simulink library "sm_trackV_lib_terrain_contact_s45"  (R2026a)
settings: Solver=VariableStepAuto
undefined symbols (not defined in the file): L1, L10, L11, L12, L13, L14, L15, L16, L17, L18, L19, L2, L20, L21, L22, L23, L24, L25, L26, L27, L28, L29, L3, L30, L31, L32, L33, L34, L35, L36, L37, L38, L39, L4, L40, L41, L42, L43, L44, L45, L5, L6, L7, L8, L9, Scene, X, Y, Z
libraries: sm_trackV_lib_terrain_contact_elem x45, $bdroot x19, sm_lib x12, sm_excv_scene_lib x3
Description:
  | Copyright 2024-2026 The MathWorks, Inc.
settings Model: Creator=smiller  LastModifiedBy=smiller

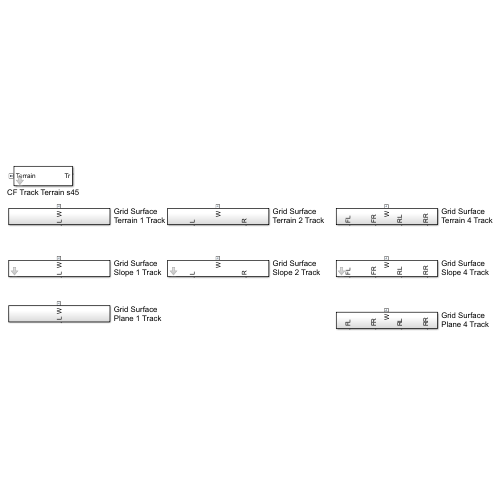
[thumbnail: Simulink's stored preview of the top-level diagram]
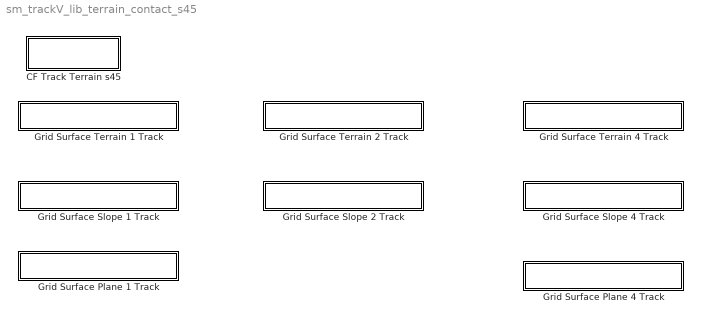
== system sm_trackV_lib_terrain_contact_s45 ==
  CF Track Terrain s45 : Subsystem  mask(Contact Forces, Full Track to Terrain){K_Road=Scene.Contact.Terrain.K, B_Road=Scene.Contact.Terrain.B, TW_Road=Scene.Contact.Terrain.TW, F_dyn_Road=Scene.Contact.Terrain.mud, F_stat_Road=Scene.Contact.Terrain.mus, CV_Road=Scene.Contact.Terrain.CV}
      mask prompts: K_Road "Normal Stiffness (N/m)"; B_Road "Normal Damping (N/(m/s))"; TW_Road "Normal Transition Width (m)"; F_dyn_Road "Coefficient of Dynamic Friction"; F_stat_Road "Coefficient of Static Friction"; CV_Road "Critical Velocity (m/s)"
      mask help: Models contact force between all track segments and the terrain.
  Grid Surface Plane 1 Track : Subsystem
  Grid Surface Plane 4 Track : Subsystem
  Grid Surface Slope 1 Track : Subsystem  mask{road_len=Scene.Slope.road_len, road_wid=Scene.Slope.road_wid, slope_rise=Scene.Slope.slope_rise, slope_run=Scene.Slope.slope_run, slope_x0=Scene.Slope.slope_start, slope_xres=Scene.Slope.slope_xres, surface_clr=Scene.Slope.clr, surface_opc=Scene.Slope.opc, K_Road=Scene.Contact.Terrain.K, B_Road=Scene.Contact.Terrain.B, TW_Road=Scene.Contact.Terrain.TW, F_dyn_Road=Scene.Contact.Terrain.mud, F_stat_Road=Scene.Contact.Terrain.mus, CV_Road=Scene.Contact.Terrain.CV}
      mask prompts: road_len "Road Length (m)"; road_wid "Road Width (m)"; slope_rise "Slope Rise (m)"; slope_run "Slope Run(m)"; slope_x0 "Slope Start (m)"; slope_xres "Slope Resolution (m)"; surface_clr "Color [R G B] (0-1)"; surface_opc "Opacity (0-1)"; K_Road "Normal Stiffness (N/m)"; B_Road "Normal Damping (N/(m/s))"; TW_Road "Normal Transition Width (m)"; F_dyn_Road "Coefficient of Dynamic Friction"; F_stat_Road "Coefficient of Static Friction"; CV_Road "Critical Velocity (m/s)"
      mask TypeOptions road_len:
      | Grid Surface
      | Slope/road_len
      mask TypeOptions road_wid:
      | Grid Surface
      | Slope/road_wid
      mask TypeOptions slope_rise:
      | Grid Surface
      | Slope/slope_rise
      mask TypeOptions slope_run:
      | Grid Surface
      | Slope/slope_run
      mask TypeOptions slope_x0:
      | Grid Surface
      | Slope/slope_x0
      mask TypeOptions slope_xres:
      | Grid Surface
      | Slope/slope_xres
      mask TypeOptions surface_clr:
      | Grid Surface
      | Slope/surface_clr
      mask TypeOptions surface_opc:
      | Grid Surface
      | Slope/surface_opc
      mask TypeOptions K_Road: CF Track Terrain L/K_Road
      mask TypeOptions B_Road: CF Track Terrain L/B_Road
      mask TypeOptions TW_Road: CF Track Terrain L/TW_Road
      mask TypeOptions F_dyn_Road: CF Track Terrain L/F_dyn_Road
      mask TypeOptions F_stat_Road: CF Track Terrain L/F_stat_Road
      mask TypeOptions CV_Road: CF Track Terrain L/CV_Road
      mask DialogControl cont_slope Prompt: Slope
      mask DialogControl cont_contact Prompt: Contact
  Grid Surface Slope 2 Track : Subsystem  mask{road_len=Scene.Slope.road_len, road_wid=Scene.Slope.road_wid, slope_rise=Scene.Slope.slope_rise, slope_run=Scene.Slope.slope_run, slope_x0=Scene.Slope.slope_start, slope_xres=Scene.Slope.slope_xres, surface_clr=Scene.Slope.clr, surface_opc=Scene.Slope.opc, K_Road=Scene.Contact.Terrain.K, B_Road=Scene.Contact.Terrain.B, TW_Road=Scene.Contact.Terrain.TW, F_dyn_Road=Scene.Contact.Terrain.mud, F_stat_Road=Scene.Contact.Terrain.mus, CV_Road=Scene.Contact.Terrain.CV}
      mask prompts: road_len "Road Length (m)"; road_wid "Road Width (m)"; slope_rise "Slope Rise (m)"; slope_run "Slope Run(m)"; slope_x0 "Slope Start (m)"; slope_xres "Slope Resolution (m)"; surface_clr "Color [R G B] (0-1)"; surface_opc "Opacity (0-1)"; K_Road "Normal Stiffness (N/m)"; B_Road "Normal Damping (N/(m/s))"; TW_Road "Normal Transition Width (m)"; F_dyn_Road "Coefficient of Dynamic Friction"; F_stat_Road "Coefficient of Static Friction"; CV_Road "Critical Velocity (m/s)"
      mask TypeOptions road_len:
      | Grid Surface
      | Slope/road_len
      mask TypeOptions road_wid:
      | Grid Surface
      | Slope/road_wid
      mask TypeOptions slope_rise:
      | Grid Surface
      | Slope/slope_rise
      mask TypeOptions slope_run:
      | Grid Surface
      | Slope/slope_run
      mask TypeOptions slope_x0:
      | Grid Surface
      | Slope/slope_x0
      mask TypeOptions slope_xres:
      | Grid Surface
      | Slope/slope_xres
      mask TypeOptions surface_clr:
      | Grid Surface
      | Slope/surface_clr
      mask TypeOptions surface_opc:
      | Grid Surface
      | Slope/surface_opc
      mask TypeOptions K_Road: CF Track Terrain L/K_Road
      mask TypeOptions B_Road: CF Track Terrain L/B_Road
      mask TypeOptions TW_Road: CF Track Terrain L/TW_Road
      mask TypeOptions F_dyn_Road: CF Track Terrain L/F_dyn_Road
      mask TypeOptions F_stat_Road: CF Track Terrain L/F_stat_Road
      mask TypeOptions CV_Road: CF Track Terrain L/CV_Road
      mask DialogControl cont_slope Prompt: Slope
      mask DialogControl cont_contact Prompt: Contact
  Grid Surface Slope 4 Track : Subsystem  mask{road_len=Scene.Slope.road_len, road_wid=Scene.Slope.road_wid, slope_rise=Scene.Slope.slope_rise, slope_run=Scene.Slope.slope_run, slope_x0=Scene.Slope.slope_start, slope_xres=Scene.Slope.slope_xres, surface_clr=Scene.Slope.clr, surface_opc=Scene.Slope.opc, K_Road=Scene.Contact.Terrain.K, B_Road=Scene.Contact.Terrain.B, TW_Road=Scene.Contact.Terrain.TW, F_dyn_Road=Scene.Contact.Terrain.mud, F_stat_Road=Scene.Contact.Terrain.mus, CV_Road=Scene.Contact.Terrain.CV}
      mask prompts: road_len "Road Length (m)"; road_wid "Road Width (m)"; slope_rise "Slope Rise (m)"; slope_run "Slope Run(m)"; slope_x0 "Slope Start (m)"; slope_xres "Slope Resolution (m)"; surface_clr "Color [R G B] (0-1)"; surface_opc "Opacity (0-1)"; K_Road "Normal Stiffness (N/m)"; B_Road "Normal Damping (N/(m/s))"; TW_Road "Normal Transition Width (m)"; F_dyn_Road "Coefficient of Dynamic Friction"; F_stat_Road "Coefficient of Static Friction"; CV_Road "Critical Velocity (m/s)"
      mask TypeOptions road_len:
      | Grid Surface
      | Slope/road_len
      mask TypeOptions road_wid:
      | Grid Surface
      | Slope/road_wid
      mask TypeOptions slope_rise:
      | Grid Surface
      | Slope/slope_rise
      mask TypeOptions slope_run:
      | Grid Surface
      | Slope/slope_run
      mask TypeOptions slope_x0:
      | Grid Surface
      | Slope/slope_x0
      mask TypeOptions slope_xres:
      | Grid Surface
      | Slope/slope_xres
      mask TypeOptions surface_clr:
      | Grid Surface
      | Slope/surface_clr
      mask TypeOptions surface_opc:
      | Grid Surface
      | Slope/surface_opc
      mask TypeOptions K_Road: CF Track Terrain FL/K_Road | CF Track Terrain FR/K_Road | CF Track Terrain RL/K_Road | CF Track Terrain RR/K_Road
      mask TypeOptions B_Road: CF Track Terrain FL/B_Road | CF Track Terrain FR/B_Road | CF Track Terrain RL/B_Road | CF Track Terrain RR/B_Road
      mask TypeOptions TW_Road: CF Track Terrain FL/TW_Road | CF Track Terrain FR/TW_Road | CF Track Terrain RL/TW_Road | CF Track Terrain RR/TW_Road
      mask TypeOptions F_dyn_Road: CF Track Terrain FL/F_dyn_Road | CF Track Terrain FR/F_dyn_Road | CF Track Terrain RL/F_dyn_Road | CF Track Terrain RR/F_dyn_Road
      mask TypeOptions F_stat_Road: CF Track Terrain FL/F_stat_Road | CF Track Terrain FR/F_stat_Road | CF Track Terrain RL/F_stat_Road | CF Track Terrain RR/F_stat_Road
      mask TypeOptions CV_Road: CF Track Terrain FL/CV_Road | CF Track Terrain FR/CV_Road | CF Track Terrain RL/CV_Road | CF Track Terrain RR/CV_Road
      mask DialogControl cont_slope Prompt: Slope
      mask DialogControl cont_contact Prompt: Contact
  Grid Surface Terrain 1 Track : Subsystem
  Grid Surface Terrain 2 Track : Subsystem
  Grid Surface Terrain 4 Track : Subsystem

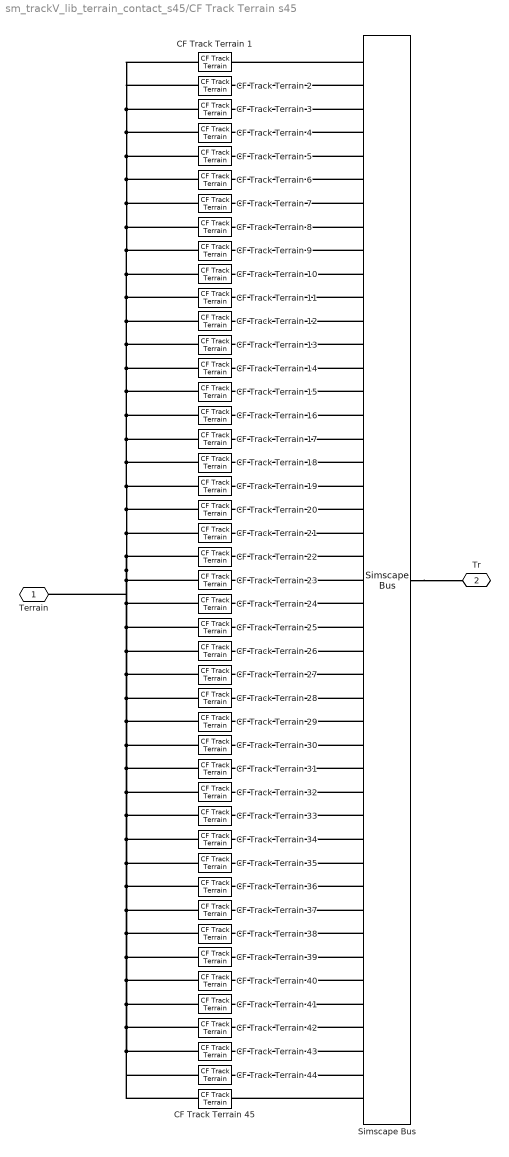
== system sm_trackV_lib_terrain_contact_s45/CF Track Terrain s45 ==
  CF Track Terrain {1..45} (45 alike) : sm_trackV_lib_terrain_contact_elem/CF Track Terrain  NormalStiffness=K_Road  NormalDamping=B_Road  NormalTransitionRegionWidth=TW_Road  CoefficientOfDynamicFriction=F_dyn_Road  CoefficientOfStaticFriction=F_stat_Road  FrictionalCriticalVelocity=CV_Road
      settings: LibrarySourceBlock=sm_chain_drive_lib/CF_Road
  Simscape Bus : SimscapeBus  HierarchyStrings=L1;L2;L3;L4;L5;L6;L7;L8;L9;L10;L11;L12;L13;L14;L15;L16;L17;L18;L19;L20;L21;L22;L23;L24;L25;L26;L27;L28;L29;L30;L31;L32;L33;L34;L35;L36;L37;L38;L39;L40;L41;L42;L43;L44;L45  ConnectionType=Bus: CBO_Seg45
  Terrain : PMIOPort  Side=Left
  Tr : PMIOPort  Port=2  Side=Right
  connections:
  CF Track Terrain 19/LConn1 -- CF Track Terrain 20/LConn1 -- CF Track Terrain 21/LConn1 -- CF Track Terrain 22/LConn1 -- CF Track Terrain 23/LConn1 -- Terrain/RConn1 -- CF Track Terrain 24/LConn1 -- CF Track Terrain 25/LConn1 -- CF Track Terrain 26/LConn1 -- CF Track Terrain 27/LConn1 -- CF Track Terrain 28/LConn1 -- CF Track Terrain 29/LConn1 -- CF Track Terrain 30/LConn1 -- CF Track Terrain 31/LConn1 -- CF Track Terrain 32/LConn1 -- CF Track Terrain 33/LConn1 -- CF Track Terrain 34/LConn1 -- CF Track Terrain 35/LConn1 -- CF Track Terrain 36/LConn1 -- CF Track Terrain 37/LConn1 -- CF Track Terrain 38/LConn1 -- CF Track Terrain 39/LConn1 -- CF Track Terrain 40/LConn1 -- CF Track Terrain 41/LConn1 -- CF Track Terrain 42/LConn1 -- CF Track Terrain 43/LConn1 -- CF Track Terrain 44/LConn1 -- CF Track Terrain 45/LConn1 -- CF Track Terrain 18/LConn1 -- CF Track Terrain 17/LConn1 -- CF Track Terrain 16/LConn1 -- CF Track Terrain 15/LConn1 -- CF Track Terrain 14/LConn1 -- CF Track Terrain 13/LConn1 -- CF Track Terrain 12/LConn1 -- CF Track Terrain 11/LConn1 -- CF Track Terrain 10/LConn1 -- CF Track Terrain 9/LConn1 -- CF Track Terrain 8/LConn1 -- CF Track Terrain 7/LConn1 -- CF Track Terrain 6/LConn1 -- CF Track Terrain 5/LConn1 -- CF Track Terrain 4/LConn1 -- CF Track Terrain 3/LConn1 -- CF Track Terrain 2/LConn1 -- CF Track Terrain 1/LConn1
  Simscape Bus/RConn1 -- Tr/RConn1
  Simscape Bus/LConn1 -- CF Track Terrain 1/RConn1
  Simscape Bus/LConn2 -- CF Track Terrain 2/RConn1
  Simscape Bus/LConn4 -- CF Track Terrain 4/RConn1
  Simscape Bus/LConn3 -- CF Track Terrain 3/RConn1
  Simscape Bus/LConn5 -- CF Track Terrain 5/RConn1
  Simscape Bus/LConn6 -- CF Track Terrain 6/RConn1
  Simscape Bus/LConn7 -- CF Track Terrain 7/RConn1
  Simscape Bus/LConn8 -- CF Track Terrain 8/RConn1
  Simscape Bus/LConn9 -- CF Track Terrain 9/RConn1
  Simscape Bus/LConn10 -- CF Track Terrain 10/RConn1
  Simscape Bus/LConn11 -- CF Track Terrain 11/RConn1
  Simscape Bus/LConn12 -- CF Track Terrain 12/RConn1
  Simscape Bus/LConn13 -- CF Track Terrain 13/RConn1
  Simscape Bus/LConn14 -- CF Track Terrain 14/RConn1
  Simscape Bus/LConn15 -- CF Track Terrain 15/RConn1
  Simscape Bus/LConn16 -- CF Track Terrain 16/RConn1
  Simscape Bus/LConn17 -- CF Track Terrain 17/RConn1
  Simscape Bus/LConn18 -- CF Track Terrain 18/RConn1
  Simscape Bus/LConn19 -- CF Track Terrain 19/RConn1
  Simscape Bus/LConn20 -- CF Track Terrain 20/RConn1
  Simscape Bus/LConn21 -- CF Track Terrain 21/RConn1
  Simscape Bus/LConn22 -- CF Track Terrain 22/RConn1
  Simscape Bus/LConn23 -- CF Track Terrain 23/RConn1
  Simscape Bus/LConn24 -- CF Track Terrain 24/RConn1
  Simscape Bus/LConn25 -- CF Track Terrain 25/RConn1
  Simscape Bus/LConn26 -- CF Track Terrain 26/RConn1
  Simscape Bus/LConn27 -- CF Track Terrain 27/RConn1
  Simscape Bus/LConn28 -- CF Track Terrain 28/RConn1
  Simscape Bus/LConn29 -- CF Track Terrain 29/RConn1
  Simscape Bus/LConn30 -- CF Track Terrain 30/RConn1
  Simscape Bus/LConn31 -- CF Track Terrain 31/RConn1
  Simscape Bus/LConn32 -- CF Track Terrain 32/RConn1
  Simscape Bus/LConn33 -- CF Track Terrain 33/RConn1
  Simscape Bus/LConn34 -- CF Track Terrain 34/RConn1
  Simscape Bus/LConn35 -- CF Track Terrain 35/RConn1
  Simscape Bus/LConn36 -- CF Track Terrain 36/RConn1
  Simscape Bus/LConn37 -- CF Track Terrain 37/RConn1
  Simscape Bus/LConn38 -- CF Track Terrain 38/RConn1
  Simscape Bus/LConn39 -- CF Track Terrain 39/RConn1
  Simscape Bus/LConn40 -- CF Track Terrain 40/RConn1
  Simscape Bus/LConn41 -- CF Track Terrain 41/RConn1
  Simscape Bus/LConn42 -- CF Track Terrain 42/RConn1
  Simscape Bus/LConn43 -- CF Track Terrain 43/RConn1
  Simscape Bus/LConn44 -- CF Track Terrain 44/RConn1
  Simscape Bus/LConn45 -- CF Track Terrain 45/RConn1

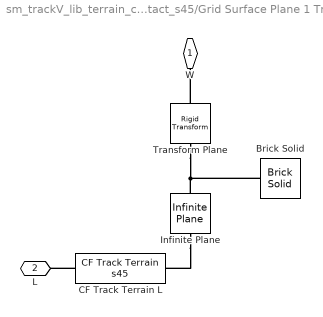
== system sm_trackV_lib_terrain_contact_s45/Grid Surface Plane 1 Track ==
  Brick Solid : sm_lib/Body Elements/Brick Solid  BrickDimensions=[28 40 0.05]  BrickDimensionsUnits=m  ExportEntireGeometry=off  InertiaType=CalculateFromGeometry  BasedOnType=Density  Density=1000  DensityUnits=kg/m^3  Mass=1  MassUnits=kg  CenterOfMass=[0 0 0]  CenterOfMassUnits=m  MomentsOfInertia=[1 1 1]  MomentsOfInertiaUnits=kg*m^2  ProductsOfInertia=[0 0 0]  ProductsOfInertiaUnits=kg*m^2  GraphicType=FromGeometry  MarkerShape=Sphere  MarkerSize=10  GraphicVisPropType=SimpleVisualProperties  GraphicDiffuseColor=[0.8196 0.7255 0.5098]  GraphicOpacity=1.0  GraphicSpecularColor=[0.5 0.5 0.5 1.0]  GraphicAmbientColor=[0.15 0.15 0.15 1.0]  GraphicEmissiveColor=[0.0 0.0 0.0 1.0]  GraphicShininess=75  DoExposeReferenceFrame=off  SerializedFrames=<Frames><Frame><Id>Frame1</Id><Value><Name>Top</Name><Origin><Source>GeometricFeature</Source><FeatureName>+z surface</FeatureName></Origin><PrimaryAxis><DefinedDirection>+Z</DefinedDirection><Source>ReferenceFrame</Source><SourceDirection>+Z</SourceDirection><FeatureName></FeatureName></PrimaryAxis><SecondaryAxis><DefinedDirection>+X</DefinedDirection><Source>ReferenceFrame</Source><SourceDirection>+X</SourceDirection><FeatureName></FeatureName></SecondaryAxis></Value></Frame></Frames>
  CF Track Terrain L : $bdroot/CF Track Terrain s45  K_Road=Scene.Contact.Terrain.K  B_Road=Scene.Contact.Terrain.B  TW_Road=Scene.Contact.Terrain.TW  F_dyn_Road=Scene.Contact.Terrain.mud  F_stat_Road=Scene.Contact.Terrain.mus  CV_Road=Scene.Contact.Terrain.CV
  Infinite Plane : sm_lib/Curves and Surfaces/Infinite Plane  GraphicType=None  GraphicPlaneWidth=28  GraphicPlaneWidthUnits=m  GraphicPlaneHeight=40  GraphicPlaneHeightUnits=m  GraphicVisPropType=SimpleVisualProperties  GraphicDiffuseColor=[0.5 0.5 0.5]  GraphicOpacity=0.25  GraphicSpecularColor=[0.5 0.5 0.5 1.0]  GraphicAmbientColor=[0.15 0.15 0.15 1.0]  GraphicEmissiveColor=[0.0 0.0 0.0 1.0]  GraphicShininess=75
  Transform Plane : sm_lib/Frames and Transforms/Rigid Transform  RotationMethod=None  FollAlignAxisA=+X  BaseAlignAxisA=+Y  FollAlignAxisB=+Y  BaseAlignAxisB=+Z  RotationStandardAxis=+Z  RotationAngle=0.0  RotationAngleUnits=deg  RotationArbitraryAxis=[0 0 1]  RotationSequenceAxes=FollowerAxes  RotationSequence=XYX  RotationSequenceAngles=[0 0 0]  RotationSequenceAnglesUnits=deg  RotationMatrix=[1 0 0; 0 1 0; 0 0 1]  Quaternion=[1 0 0 0]  TranslationMethod=Cartesian  TranslationCartesianOffset=[1.5 17*0 0]  TranslationCartesianOffsetUnits=m  TranslationStandardAxis=+Z  TranslationStandardOffset=0  TranslationStandardOffsetUnits=m  TranslationROffset=0  TranslationROffsetUnits=m  TranslationThetaOffset=0  TranslationThetaOffsetUnits=deg  TranslationZOffset=0  TranslationZOffsetUnits=m
  W : PMIOPort  Side=Right
  L : PMIOPort  Port=2  Side=Left
  connections:
  Transform Plane/LConn1 -- W/RConn1
  Infinite Plane/RConn1 -- CF Track Terrain L/LConn1
  Infinite Plane/LConn1 -- Transform Plane/RConn1 -- Brick Solid/LConn1
  CF Track Terrain L/RConn1 -- L/RConn1

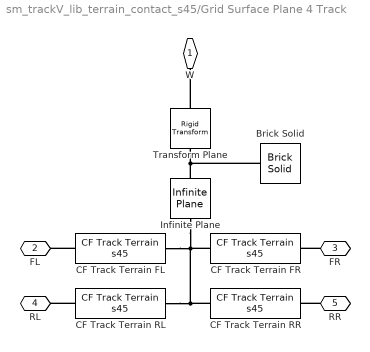
== system sm_trackV_lib_terrain_contact_s45/Grid Surface Plane 4 Track ==
  Brick Solid : sm_lib/Body Elements/Brick Solid  BrickDimensions=[28 40 0.05]  BrickDimensionsUnits=m  ExportEntireGeometry=off  InertiaType=CalculateFromGeometry  BasedOnType=Density  Density=1000  DensityUnits=kg/m^3  Mass=1  MassUnits=kg  CenterOfMass=[0 0 0]  CenterOfMassUnits=m  MomentsOfInertia=[1 1 1]  MomentsOfInertiaUnits=kg*m^2  ProductsOfInertia=[0 0 0]  ProductsOfInertiaUnits=kg*m^2  GraphicType=FromGeometry  MarkerShape=Sphere  MarkerSize=10  GraphicVisPropType=SimpleVisualProperties  GraphicDiffuseColor=[0.8196 0.7255 0.5098]  GraphicOpacity=1.0  GraphicSpecularColor=[0.5 0.5 0.5 1.0]  GraphicAmbientColor=[0.15 0.15 0.15 1.0]  GraphicEmissiveColor=[0.0 0.0 0.0 1.0]  GraphicShininess=75  DoExposeReferenceFrame=off  SerializedFrames=<Frames><Frame><Id>Frame1</Id><Value><Name>Top</Name><Origin><Source>GeometricFeature</Source><FeatureName>+z surface</FeatureName></Origin><PrimaryAxis><DefinedDirection>+Z</DefinedDirection><Source>ReferenceFrame</Source><SourceDirection>+Z</SourceDirection><FeatureName></FeatureName></PrimaryAxis><SecondaryAxis><DefinedDirection>+X</DefinedDirection><Source>ReferenceFrame</Source><SourceDirection>+X</SourceDirection><FeatureName></FeatureName></SecondaryAxis></Value></Frame></Frames>
  CF Track Terrain FL : $bdroot/CF Track Terrain s45  K_Road=Scene.Contact.Terrain.K  B_Road=Scene.Contact.Terrain.B  TW_Road=Scene.Contact.Terrain.TW  F_dyn_Road=Scene.Contact.Terrain.mud  F_stat_Road=Scene.Contact.Terrain.mus  CV_Road=Scene.Contact.Terrain.CV
  CF Track Terrain FR : $bdroot/CF Track Terrain s45  K_Road=Scene.Contact.Terrain.K  B_Road=Scene.Contact.Terrain.B  TW_Road=Scene.Contact.Terrain.TW  F_dyn_Road=Scene.Contact.Terrain.mud  F_stat_Road=Scene.Contact.Terrain.mus  CV_Road=Scene.Contact.Terrain.CV
  CF Track Terrain RL : $bdroot/CF Track Terrain s45  K_Road=Scene.Contact.Terrain.K  B_Road=Scene.Contact.Terrain.B  TW_Road=Scene.Contact.Terrain.TW  F_dyn_Road=Scene.Contact.Terrain.mud  F_stat_Road=Scene.Contact.Terrain.mus  CV_Road=Scene.Contact.Terrain.CV
  CF Track Terrain RR : $bdroot/CF Track Terrain s45  K_Road=Scene.Contact.Terrain.K  B_Road=Scene.Contact.Terrain.B  TW_Road=Scene.Contact.Terrain.TW  F_dyn_Road=Scene.Contact.Terrain.mud  F_stat_Road=Scene.Contact.Terrain.mus  CV_Road=Scene.Contact.Terrain.CV
  Infinite Plane : sm_lib/Curves and Surfaces/Infinite Plane  GraphicType=None  GraphicPlaneWidth=28  GraphicPlaneWidthUnits=m  GraphicPlaneHeight=40  GraphicPlaneHeightUnits=m  GraphicVisPropType=SimpleVisualProperties  GraphicDiffuseColor=[0.5 0.5 0.5]  GraphicOpacity=0.25  GraphicSpecularColor=[0.5 0.5 0.5 1.0]  GraphicAmbientColor=[0.15 0.15 0.15 1.0]  GraphicEmissiveColor=[0.0 0.0 0.0 1.0]  GraphicShininess=75
  Transform Plane : sm_lib/Frames and Transforms/Rigid Transform  RotationMethod=None  FollAlignAxisA=+X  BaseAlignAxisA=+Y  FollAlignAxisB=+Y  BaseAlignAxisB=+Z  RotationStandardAxis=+Z  RotationAngle=0.0  RotationAngleUnits=deg  RotationArbitraryAxis=[0 0 1]  RotationSequenceAxes=FollowerAxes  RotationSequence=XYX  RotationSequenceAngles=[0 0 0]  RotationSequenceAnglesUnits=deg  RotationMatrix=[1 0 0; 0 1 0; 0 0 1]  Quaternion=[1 0 0 0]  TranslationMethod=Cartesian  TranslationCartesianOffset=[1.5 17 0]  TranslationCartesianOffsetUnits=m  TranslationStandardAxis=+Z  TranslationStandardOffset=0  TranslationStandardOffsetUnits=m  TranslationROffset=0  TranslationROffsetUnits=m  TranslationThetaOffset=0  TranslationThetaOffsetUnits=deg  TranslationZOffset=0  TranslationZOffsetUnits=m
  W : PMIOPort  Side=Right
  FL : PMIOPort  Port=2  Side=Left
  FR : PMIOPort  Port=3  Side=Left
  RL : PMIOPort  Port=4  Side=Left
  RR : PMIOPort  Port=5  Side=Left
  connections:
  Transform Plane/RConn1 -- Brick Solid/LConn1 -- Infinite Plane/LConn1
  FR/RConn1 -- CF Track Terrain FR/RConn1
  Transform Plane/LConn1 -- W/RConn1
  CF Track Terrain RR/LConn1 -- CF Track Terrain FR/LConn1 -- CF Track Terrain FL/LConn1 -- Infinite Plane/RConn1 -- CF Track Terrain RL/LConn1
  CF Track Terrain FL/RConn1 -- FL/RConn1
  CF Track Terrain RL/RConn1 -- RL/RConn1
  RR/RConn1 -- CF Track Terrain RR/RConn1

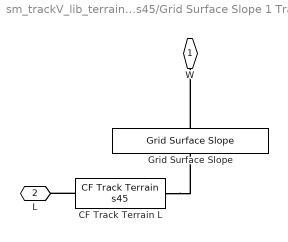
== system sm_trackV_lib_terrain_contact_s45/Grid Surface Slope 1 Track ==
  CF Track Terrain L : $bdroot/CF Track Terrain s45  K_Road=K_Road  B_Road=B_Road  TW_Road=TW_Road  F_dyn_Road=F_dyn_Road  F_stat_Road=F_stat_Road  CV_Road=CV_Road
  Grid Surface Slope : sm_excv_scene_lib/Grid Surface Slope  road_len=road_len  road_wid=road_wid  slope_run=slope_run  slope_rise=slope_rise  slope_x0=slope_x0  slope_xres=slope_xres  surface_clr=surface_clr  surface_opc=surface_opc
  W : PMIOPort  Side=Right
  L : PMIOPort  Port=2  Side=Left
  connections:
  CF Track Terrain L/LConn1 -- Grid Surface Slope/LConn1
  Grid Surface Slope/RConn1 -- W/RConn1
  CF Track Terrain L/RConn1 -- L/RConn1

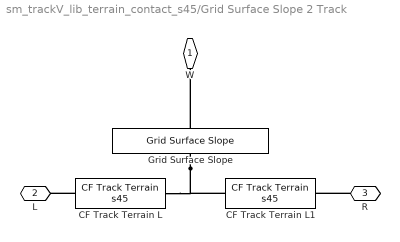
== system sm_trackV_lib_terrain_contact_s45/Grid Surface Slope 2 Track ==
  CF Track Terrain L : $bdroot/CF Track Terrain s45  K_Road=K_Road  B_Road=B_Road  TW_Road=TW_Road  F_dyn_Road=F_dyn_Road  F_stat_Road=F_stat_Road  CV_Road=CV_Road
  CF Track Terrain L1 : $bdroot/CF Track Terrain s45  K_Road=K_Road  B_Road=B_Road  TW_Road=TW_Road  F_dyn_Road=F_dyn_Road  F_stat_Road=F_stat_Road  CV_Road=CV_Road
  Grid Surface Slope : sm_excv_scene_lib/Grid Surface Slope  road_len=road_len  road_wid=road_wid  slope_run=slope_run  slope_rise=slope_rise  slope_x0=slope_x0  slope_xres=slope_xres  surface_clr=surface_clr  surface_opc=surface_opc
  W : PMIOPort  Side=Right
  L : PMIOPort  Port=2  Side=Left
  R : PMIOPort  Port=3  Side=Left
  connections:
  R/RConn1 -- CF Track Terrain L1/RConn1
  CF Track Terrain L/RConn1 -- L/RConn1
  Grid Surface Slope/RConn1 -- W/RConn1
  Grid Surface Slope/LConn1 -- CF Track Terrain L1/LConn1 -- CF Track Terrain L/LConn1

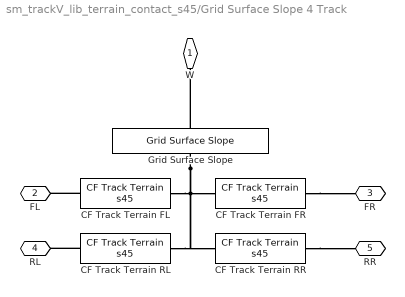
== system sm_trackV_lib_terrain_contact_s45/Grid Surface Slope 4 Track ==
  CF Track Terrain FL : $bdroot/CF Track Terrain s45  K_Road=K_Road  B_Road=B_Road  TW_Road=TW_Road  F_dyn_Road=F_dyn_Road  F_stat_Road=F_stat_Road  CV_Road=CV_Road
  CF Track Terrain FR : $bdroot/CF Track Terrain s45  K_Road=K_Road  B_Road=B_Road  TW_Road=TW_Road  F_dyn_Road=F_dyn_Road  F_stat_Road=F_stat_Road  CV_Road=CV_Road
  CF Track Terrain RL : $bdroot/CF Track Terrain s45  K_Road=K_Road  B_Road=B_Road  TW_Road=TW_Road  F_dyn_Road=F_dyn_Road  F_stat_Road=F_stat_Road  CV_Road=CV_Road
  CF Track Terrain RR : $bdroot/CF Track Terrain s45  K_Road=K_Road  B_Road=B_Road  TW_Road=TW_Road  F_dyn_Road=F_dyn_Road  F_stat_Road=F_stat_Road  CV_Road=CV_Road
  Grid Surface Slope : sm_excv_scene_lib/Grid Surface Slope  road_len=road_len  road_wid=road_wid  slope_run=slope_run  slope_rise=slope_rise  slope_x0=slope_x0  slope_xres=slope_xres  surface_clr=surface_clr  surface_opc=surface_opc
  W : PMIOPort  Side=Right
  FL : PMIOPort  Port=2  Side=Left
  FR : PMIOPort  Port=3  Side=Left
  RL : PMIOPort  Port=4  Side=Left
  RR : PMIOPort  Port=5  Side=Left
  connections:
  CF Track Terrain FR/RConn1 -- FR/RConn1
  CF Track Terrain FL/RConn1 -- FL/RConn1
  Grid Surface Slope/RConn1 -- W/RConn1
  Grid Surface Slope/LConn1 -- CF Track Terrain FR/LConn1 -- CF Track Terrain FL/LConn1 -- CF Track Terrain RR/LConn1 -- CF Track Terrain RL/LConn1
  CF Track Terrain RL/RConn1 -- RL/RConn1
  CF Track Terrain RR/RConn1 -- RR/RConn1

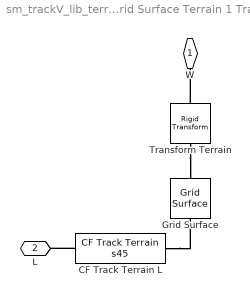
== system sm_trackV_lib_terrain_contact_s45/Grid Surface Terrain 1 Track ==
  CF Track Terrain L : $bdroot/CF Track Terrain s45  K_Road=Scene.Contact.Terrain.K  B_Road=Scene.Contact.Terrain.B  TW_Road=Scene.Contact.Terrain.TW  F_dyn_Road=Scene.Contact.Terrain.mud  F_stat_Road=Scene.Contact.Terrain.mus  CV_Road=Scene.Contact.Terrain.CV
  Grid Surface : sm_lib/Curves and Surfaces/Grid Surface  XGridVector=Scene.Terrain.xg  XGridVectorUnits=m  YGridVector=Scene.Terrain.yg  YGridVectorUnits=m  ZHeights=Scene.Terrain.z_heights_data  ZHeightsUnits=m  GraphicType=FromGeometry  GraphicVisPropType=SimpleVisualProperties  GraphicDiffuseColor=[0.8196 0.7255 0.5098]  GraphicOpacity=1.0  GraphicSpecularColor=[0.5 0.5 0.5 1.0]  GraphicAmbientColor=[0.15 0.15 0.15 1.0]  GraphicEmissiveColor=[0.0 0.0 0.0 1.0]  GraphicShininess=75
  Transform Terrain : sm_lib/Frames and Transforms/Rigid Transform  RotationMethod=None  FollAlignAxisA=+X  BaseAlignAxisA=+Y  FollAlignAxisB=+Y  BaseAlignAxisB=+Z  RotationStandardAxis=+Z  RotationAngle=0.0  RotationAngleUnits=deg  RotationArbitraryAxis=[0 0 1]  RotationSequenceAxes=FollowerAxes  RotationSequence=XYX  RotationSequenceAngles=[0 0 0]  RotationSequenceAnglesUnits=deg  RotationMatrix=[1 0 0; 0 1 0; 0 0 1]  Quaternion=[1 0 0 0]  TranslationMethod=Cartesian  TranslationCartesianOffset="[-45 -45+2.5  -2.75+0.2]"  TranslationCartesianOffsetUnits=m  TranslationStandardAxis=+Z  TranslationStandardOffset=0  TranslationStandardOffsetUnits=m  TranslationROffset=0  TranslationROffsetUnits=m  TranslationThetaOffset=0  TranslationThetaOffsetUnits=deg  TranslationZOffset=0  TranslationZOffsetUnits=m
  W : PMIOPort  Side=Right
  L : PMIOPort  Port=2  Side=Left
  connections:
  CF Track Terrain L/RConn1 -- L/RConn1
  Transform Terrain/RConn1 -- Grid Surface/LConn1
  CF Track Terrain L/LConn1 -- Grid Surface/RConn1
  Transform Terrain/LConn1 -- W/RConn1

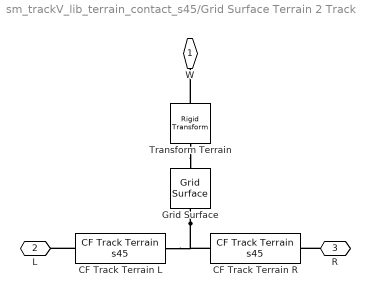
== system sm_trackV_lib_terrain_contact_s45/Grid Surface Terrain 2 Track ==
  CF Track Terrain L : $bdroot/CF Track Terrain s45  K_Road=Scene.Contact.Terrain.K  B_Road=Scene.Contact.Terrain.B  TW_Road=Scene.Contact.Terrain.TW  F_dyn_Road=Scene.Contact.Terrain.mud  F_stat_Road=Scene.Contact.Terrain.mus  CV_Road=Scene.Contact.Terrain.CV
  CF Track Terrain R : $bdroot/CF Track Terrain s45  K_Road=Scene.Contact.Terrain.K  B_Road=Scene.Contact.Terrain.B  TW_Road=Scene.Contact.Terrain.TW  F_dyn_Road=Scene.Contact.Terrain.mud  F_stat_Road=Scene.Contact.Terrain.mus  CV_Road=Scene.Contact.Terrain.CV
  Grid Surface : sm_lib/Curves and Surfaces/Grid Surface  XGridVector=Scene.Terrain.xg  XGridVectorUnits=m  YGridVector=Scene.Terrain.yg  YGridVectorUnits=m  ZHeights=Scene.Terrain.z_heights_data  ZHeightsUnits=m  GraphicType=FromGeometry  GraphicVisPropType=SimpleVisualProperties  GraphicDiffuseColor=[0.8196 0.7255 0.5098]  GraphicOpacity=1.0  GraphicSpecularColor=[0.5 0.5 0.5 1.0]  GraphicAmbientColor=[0.15 0.15 0.15 1.0]  GraphicEmissiveColor=[0.0 0.0 0.0 1.0]  GraphicShininess=75
  Transform Terrain : sm_lib/Frames and Transforms/Rigid Transform  RotationMethod=None  FollAlignAxisA=+X  BaseAlignAxisA=+Y  FollAlignAxisB=+Y  BaseAlignAxisB=+Z  RotationStandardAxis=+Z  RotationAngle=0.0  RotationAngleUnits=deg  RotationArbitraryAxis=[0 0 1]  RotationSequenceAxes=FollowerAxes  RotationSequence=XYX  RotationSequenceAngles=[0 0 0]  RotationSequenceAnglesUnits=deg  RotationMatrix=[1 0 0; 0 1 0; 0 0 1]  Quaternion=[1 0 0 0]  TranslationMethod=Cartesian  TranslationCartesianOffset="[-45 -45+2.5  -2.75+0.2]"  TranslationCartesianOffsetUnits=m  TranslationStandardAxis=+Z  TranslationStandardOffset=0  TranslationStandardOffsetUnits=m  TranslationROffset=0  TranslationROffsetUnits=m  TranslationThetaOffset=0  TranslationThetaOffsetUnits=deg  TranslationZOffset=0  TranslationZOffsetUnits=m
  W : PMIOPort  Side=Right
  L : PMIOPort  Port=2  Side=Left
  R : PMIOPort  Port=3  Side=Left
  connections:
  R/RConn1 -- CF Track Terrain R/RConn1
  Transform Terrain/LConn1 -- W/RConn1
  Grid Surface/RConn1 -- CF Track Terrain R/LConn1 -- CF Track Terrain L/LConn1
  Transform Terrain/RConn1 -- Grid Surface/LConn1
  CF Track Terrain L/RConn1 -- L/RConn1

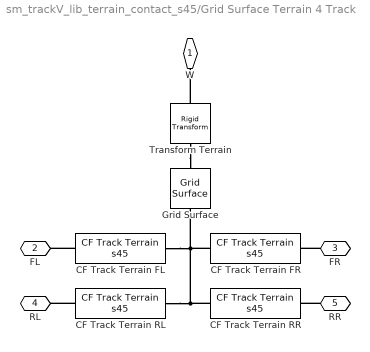
== system sm_trackV_lib_terrain_contact_s45/Grid Surface Terrain 4 Track ==
  CF Track Terrain FL : $bdroot/CF Track Terrain s45  K_Road=Scene.Contact.Terrain.K  B_Road=Scene.Contact.Terrain.B  TW_Road=Scene.Contact.Terrain.TW  F_dyn_Road=Scene.Contact.Terrain.mud  F_stat_Road=Scene.Contact.Terrain.mus  CV_Road=Scene.Contact.Terrain.CV
  CF Track Terrain FR : $bdroot/CF Track Terrain s45  K_Road=Scene.Contact.Terrain.K  B_Road=Scene.Contact.Terrain.B  TW_Road=Scene.Contact.Terrain.TW  F_dyn_Road=Scene.Contact.Terrain.mud  F_stat_Road=Scene.Contact.Terrain.mus  CV_Road=Scene.Contact.Terrain.CV
  CF Track Terrain RL : $bdroot/CF Track Terrain s45  K_Road=Scene.Contact.Terrain.K  B_Road=Scene.Contact.Terrain.B  TW_Road=Scene.Contact.Terrain.TW  F_dyn_Road=Scene.Contact.Terrain.mud  F_stat_Road=Scene.Contact.Terrain.mus  CV_Road=Scene.Contact.Terrain.CV
  CF Track Terrain RR : $bdroot/CF Track Terrain s45  K_Road=Scene.Contact.Terrain.K  B_Road=Scene.Contact.Terrain.B  TW_Road=Scene.Contact.Terrain.TW  F_dyn_Road=Scene.Contact.Terrain.mud  F_stat_Road=Scene.Contact.Terrain.mus  CV_Road=Scene.Contact.Terrain.CV
  Grid Surface : sm_lib/Curves and Surfaces/Grid Surface  XGridVector=Scene.Terrain.xg  XGridVectorUnits=m  YGridVector=Scene.Terrain.yg  YGridVectorUnits=m  ZHeights=Scene.Terrain.z_heights_data  ZHeightsUnits=m  GraphicType=FromGeometry  GraphicVisPropType=SimpleVisualProperties  GraphicDiffuseColor=[0.8196 0.7255 0.5098]  GraphicOpacity=1.0  GraphicSpecularColor=[0.5 0.5 0.5 1.0]  GraphicAmbientColor=[0.15 0.15 0.15 1.0]  GraphicEmissiveColor=[0.0 0.0 0.0 1.0]  GraphicShininess=75
  Transform Terrain : sm_lib/Frames and Transforms/Rigid Transform  RotationMethod=None  FollAlignAxisA=+X  BaseAlignAxisA=+Y  FollAlignAxisB=+Y  BaseAlignAxisB=+Z  RotationStandardAxis=+Z  RotationAngle=0.0  RotationAngleUnits=deg  RotationArbitraryAxis=[0 0 1]  RotationSequenceAxes=FollowerAxes  RotationSequence=XYX  RotationSequenceAngles=[0 0 0]  RotationSequenceAnglesUnits=deg  RotationMatrix=[1 0 0; 0 1 0; 0 0 1]  Quaternion=[1 0 0 0]  TranslationMethod=Cartesian  TranslationCartesianOffset="[-45 -45+2.5  -2.75+0.2]"  TranslationCartesianOffsetUnits=m  TranslationStandardAxis=+Z  TranslationStandardOffset=0  TranslationStandardOffsetUnits=m  TranslationROffset=0  TranslationROffsetUnits=m  TranslationThetaOffset=0  TranslationThetaOffsetUnits=deg  TranslationZOffset=0  TranslationZOffsetUnits=m
  W : PMIOPort  Side=Right
  FL : PMIOPort  Port=2  Side=Left
  FR : PMIOPort  Port=3  Side=Left
  RL : PMIOPort  Port=4  Side=Left
  RR : PMIOPort  Port=5  Side=Left
  connections:
  RR/RConn1 -- CF Track Terrain RR/RConn1
  CF Track Terrain RL/RConn1 -- RL/RConn1
  CF Track Terrain FL/RConn1 -- FL/RConn1
  Transform Terrain/RConn1 -- Grid Surface/LConn1
  CF Track Terrain RL/LConn1 -- CF Track Terrain FL/LConn1 -- CF Track Terrain FR/LConn1 -- Grid Surface/RConn1 -- CF Track Terrain RR/LConn1
  Transform Terrain/LConn1 -- W/RConn1
  FR/RConn1 -- CF Track Terrain FR/RConn1
